simulink model "assignment_13_force_control_inner_position_2"  (R2022b)
settings: Solver=VariableStepAuto  StartTime=0.0  StopTime=5  RelTol=1e-3
values from neighbouring files (symbols this model uses):
  dq0 = [0;0;0]    [assignment_10.m]    (also in assignment_11.m; assignment_12.m; assignment_13.m; assignment_6.m)
  Fd = [0; 0; 3]    [assignment_13.m]
  K_env = 1000    [assignment_11.m]    (also in assignment_12.m = 100; assignment_13.m = 100)
  Kd_pos = 10    [assignment_13.m]
  Ki_force = 0.1    [assignment_13.m]
  Kp_force = 1    [assignment_13.m]
  Kp_pos = 10    [assignment_13.m]
  q0 = [0;0;0]    [assignment_10.m]    (also in assignment_11.m; assignment_12.m; assignment_13.m = [0; pi/2; -pi/2]; assignment_6.m)
  x_home = direct_kinematics(q_home)    [assignment_11.m]    (also in assignment_13.m = x_home(1:3, 1))
  x_ref = x_rest_env    [assignment_13.m]
  x_rest_env = direct_kinematics(q_rest_env)    [assignment_11.m]    (also in assignment_12.m; assignment_13.m = x_rest_env(1:3, 1))
settings Model: Creator=acesi  LastModifiedBy=Manu

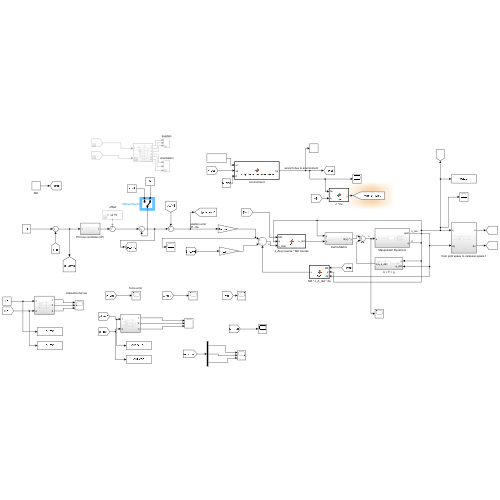
[thumbnail: Simulink's stored preview of the top-level diagram]
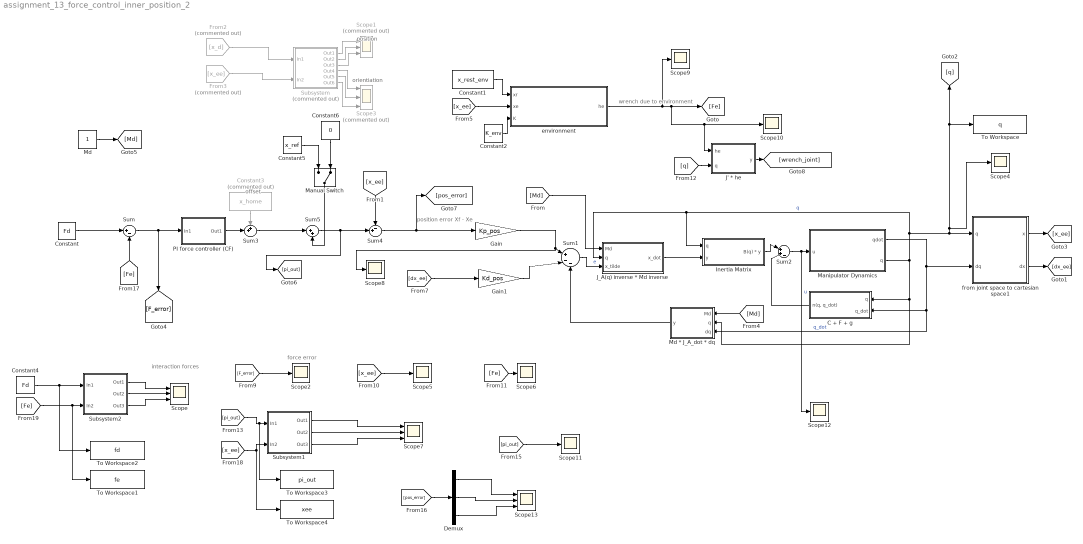
== system assignment_13_force_control_inner_position_2 ==
  note: force error
  note: interaction forces
  note: position error
      | Xf - Xe
  note: offset
  note: orientiation
  note: position
  note: wrench due to environment
  C + F + g : Subsystem
  Constant : Constant  Value=Fd
  Constant1 : Constant  Value=x_rest_env
  Constant2 : Constant  Value=K_env
  Constant3 : Constant  Commented=on  Value=x_home
  Constant4 : Constant  Value=Fd
  Constant5 : Constant  Value=x_ref
  Constant6 : Constant  Value=0
  Demux : Demux  Outputs=3
  From2 : From  Commented=on  GotoTag=x_d
  From3 : From  Commented=on  GotoTag=x_ee
  Gain : Gain  Gain=Kp_pos
  Gain1 : Gain  Gain=Kd_pos
  Inertia Matrix : Subsystem
  J' * he : MATLAB Function  TreatAsAtomicUnit=on
  J_A(q) inverse * Md inverse : MATLAB Function  TreatAsAtomicUnit=on
  Manipulator Dynamics : Subsystem
  Manual Switch : ManualSwitch  CurrentSetting=0
  Md : Constant
  Md * J_A_dot * dq : MATLAB Function  TreatAsAtomicUnit=on
  PI force controller (CF) : Subsystem
  Scope : Scope  NumInputPorts=3
  Scope1 : Scope  Commented=on  NumInputPorts=3
  Scope{2,4..6,8..12} (9 alike) : Scope
  Scope13 : Scope  NumInputPorts=3
  Scope3 : Scope  Commented=on  NumInputPorts=3
  Scope7 : Scope  NumInputPorts=3
  Subsystem : Subsystem  Commented=on
  Subsystem1 : Subsystem
  Subsystem2 : Subsystem
  Sum : Sum  Inputs=|+-
  Sum1 : Sum  Inputs=|+--
  Sum2 : Sum  Inputs=|++-
  Sum3 : Sum  Inputs=++|
  Sum4 : Sum  Inputs=-+|
  Sum5 : Sum  Inputs=|++
  To Workspace : ToWorkspace  VariableName=q  SaveFormat=Timeseries  SampleTime=-1
  To Workspace1 : ToWorkspace  VariableName=fe  SaveFormat=Timeseries  SampleTime=-1
  To Workspace2 : ToWorkspace  VariableName=fd  SaveFormat=Timeseries  SampleTime=-1
  To Workspace3 : ToWorkspace  VariableName=pi_out  SaveFormat=Timeseries  SampleTime=-1
  To Workspace4 : ToWorkspace  VariableName=xee  SaveFormat=Timeseries  SampleTime=-1
  environment : MATLAB Function  TreatAsAtomicUnit=on
  from joint space to cartesian space1 : Subsystem
  wires:
  Manipulator Dynamics/1(qdot) -> from joint space to cartesian space1/2(dq), Md * J_A_dot * dq/3(dq), C + F + g/2(q_dot)  "q_dot"
  Manipulator Dynamics/2(q) -> J_A(q) inverse * Md inverse/2(q), Inertia Matrix/1(q), from joint space to cartesian space1/1(q), Scope4/1, To Workspace/1, [q], Md * J_A_dot * dq/2(q), C + F + g/1(q)  "q"
  Inertia Matrix/1(B(q) * y) -> Sum2/1
  Sum2/1 -> Scope12/1, Manipulator Dynamics/1(u)  "u"
  C + F + g/1("n(q, q_dot)") -> Sum2/2
  Sum1/1 -> J_A(q) inverse * Md inverse/3(x_tilde)  "e"
  J_A(q) inverse * Md inverse/1(x_dot) -> Inertia Matrix/2(y)
  From2/1 -> Subsystem/1(In1)
  From3/1 -> Subsystem/2(In2)
  Subsystem/6(Out6) -> Scope3/3
  Subsystem/2(Out2) -> Scope1/2
  Subsystem/4(Out4) -> Scope3/1
  Subsystem/3(Out3) -> Scope1/3
  Subsystem/5(Out5) -> Scope3/2
  Subsystem/1(Out1) -> Scope1/1
  [Md] -> J_A(q) inverse * Md inverse/1(Md)
  Md/1 -> [Md]
  [Md] -> Md * J_A_dot * dq/1(Md)
  Constant2/1 -> environment/3(K)
  [x_ee] -> environment/2(xe)
  Constant1/1 -> environment/1(xr)
  environment/1(he) -> Scope9/1, Scope10/1, J' * he/1(he), [Fe]
  from joint space to cartesian space1/1(x) -> [x_ee]
  from joint space to cartesian space1/2(dx) -> [dx_ee]
  PI force controller (CF)/1(Out1) -> Sum3/2
  Sum/1 -> PI force controller (CF)/1(In1), [F_error]
  [x_ee] -> Sum4/1
  Sum4/1 -> [pos_error], Gain/1
  Md * J_A_dot * dq/1(y) -> Sum1/3
  [Fe] -> Sum/2
  [F_error] -> Scope2/1
  [x_ee] -> Scope5/1
  [dx_ee] -> Gain1/1
  Gain1/1 -> Sum1/2
  [Fe] -> Scope6/1
  [q] -> J' * he/2(q)
  Gain/1 -> Scope8/1, Sum1/1
  [pi_out] -> To Workspace3/1, Subsystem1/1(In1)
  Subsystem1/1(Out1) -> Scope7/1
  [x_ee] -> To Workspace4/1, Subsystem1/2(In2)
  Subsystem1/2(Out2) -> Scope7/2
  Subsystem1/3(Out3) -> Scope7/3
  [pi_out] -> Scope11/1
  J' * he/1(y) -> [wrench_joint]
  Demux/3 -> Scope13/3
  Demux/1 -> Scope13/1
  [pos_error] -> Demux/1
  Demux/2 -> Scope13/2
  Sum3/1 -> Sum5/1
  [Fe] -> Subsystem2/2(In2), To Workspace1/1
  Constant4/1 -> Subsystem2/1(In1), To Workspace2/1
  Subsystem2/1(Out1) -> Scope/1
  Subsystem2/2(Out2) -> Scope/2
  Subsystem2/3(Out3) -> Scope/3
  Constant/1 -> Sum/1
  Constant3/1 -> Sum3/1
  Constant5/1 -> Manual Switch/1
  Constant6/1 -> Manual Switch/2
  Sum5/1 -> [pi_out], Sum4/2
  Manual Switch/1 -> Sum5/2

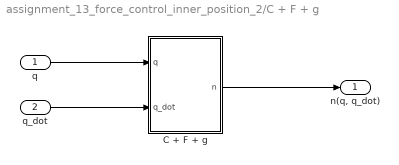
== system assignment_13_force_control_inner_position_2/C + F + g ==
  q : Inport
  q_dot : Inport  Port=2
  C + F + g : MATLAB Function  TreatAsAtomicUnit=on
  "n(q, q_dot)" : Outport
  wires:
  C + F + g/1(n) -> "n(q, q_dot)"/1
  q/1 -> C + F + g/1(q)
  q_dot/1 -> C + F + g/2(q_dot)

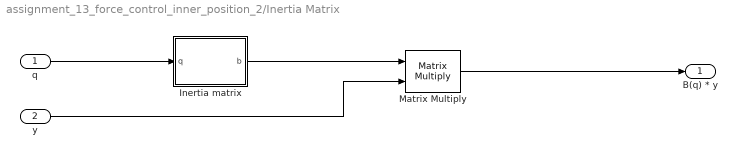
== system assignment_13_force_control_inner_position_2/Inertia Matrix ==
  q : Inport
  y : Inport  Port=2
  Inertia matrix : MATLAB Function  TreatAsAtomicUnit=on
  Matrix Multiply : Product  Multiplication=Matrix(*)
  B(q) * y : Outport
  wires:
  q/1 -> Inertia matrix/1(q)
  Inertia matrix/1(b) -> Matrix Multiply/1
  y/1 -> Matrix Multiply/2
  Matrix Multiply/1 -> B(q) * y/1

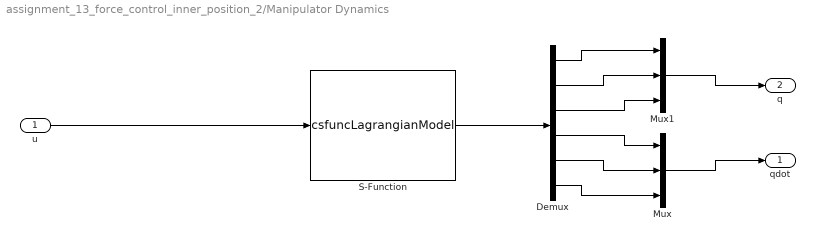
== system assignment_13_force_control_inner_position_2/Manipulator Dynamics ==
  u : Inport
  Demux : Demux  Outputs=6
  Mux : Mux  Inputs=3
  Mux1 : Mux  Inputs=3
  S-Function : S-Function  FunctionName=csfuncLagrangianModel  Parameters=q0 dq0  SFunctionDeploymentMode=off  EnableBusSupport=off
  qdot : Outport
  q : Outport  Port=2
  wires:
  u/1 -> S-Function/1
  S-Function/1 -> Demux/1
  Mux1/1 -> q/1
  Mux/1 -> qdot/1
  Demux/6 -> Mux/3
  Demux/5 -> Mux/2
  Demux/4 -> Mux/1
  Demux/3 -> Mux1/3
  Demux/2 -> Mux1/2
  Demux/1 -> Mux1/1

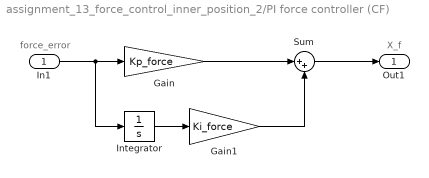
== system assignment_13_force_control_inner_position_2/PI force controller (CF) ==
  note: X_f
  note: force_error
  In1 : Inport
  Gain : Gain  Gain=Kp_force
  Gain1 : Gain  Gain=Ki_force
  Integrator : Integrator
  Sum : Sum  Inputs=|++
  Out1 : Outport
  wires:
  In1/1 -> Integrator/1, Gain/1
  Sum/1 -> Out1/1
  Gain/1 -> Sum/1
  Gain1/1 -> Sum/2
  Integrator/1 -> Gain1/1

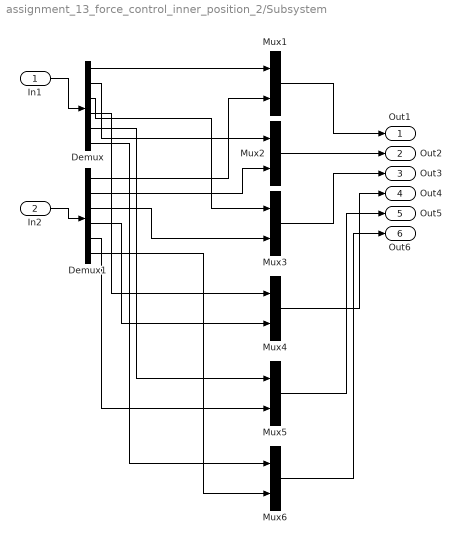
== system assignment_13_force_control_inner_position_2/Subsystem ==
  In1 : Inport
  In2 : Inport  Port=2
  Demux : Demux  Outputs=6
  Demux1 : Demux  Outputs=6
  Mux{1..6} (6 alike) : Mux  Inputs=2
  Out1 : Outport
  Out2 : Outport  Port=2
  Out3 : Outport  Port=3
  Out4 : Outport  Port=4
  Out5 : Outport  Port=5
  Out6 : Outport  Port=6
  wires:
  Demux/1 -> Mux1/1
  Demux/3 -> Mux3/1
  Demux/2 -> Mux2/1
  Demux1/1 -> Mux1/2
  Mux2/1 -> Out2/1
  Demux1/3 -> Mux3/2
  Demux1/2 -> Mux2/2
  Mux3/1 -> Out3/1
  Mux1/1 -> Out1/1
  In2/1 -> Demux1/1
  In1/1 -> Demux/1
  Demux1/4 -> Mux4/2
  Demux/4 -> Mux4/1
  Demux/5 -> Mux5/1
  Demux1/5 -> Mux5/2
  Demux/6 -> Mux6/1
  Demux1/6 -> Mux6/2
  Mux4/1 -> Out4/1
  Mux5/1 -> Out5/1
  Mux6/1 -> Out6/1

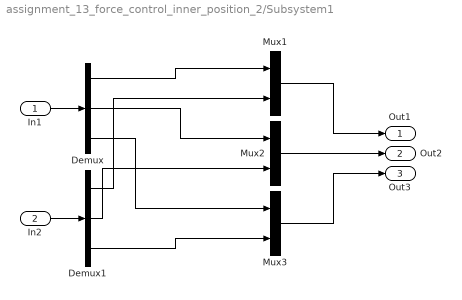
== system assignment_13_force_control_inner_position_2/Subsystem1 ==
  In1 : Inport
  In2 : Inport  Port=2
  Demux : Demux  Outputs=3
  Demux1 : Demux  Outputs=3
  Mux1 : Mux  Inputs=2
  Mux2 : Mux  Inputs=2
  Mux3 : Mux  Inputs=2
  Out1 : Outport
  Out2 : Outport  Port=2
  Out3 : Outport  Port=3
  wires:
  Mux2/1 -> Out2/1
  Mux3/1 -> Out3/1
  Mux1/1 -> Out1/1
  In2/1 -> Demux1/1
  In1/1 -> Demux/1
  Demux/1 -> Mux1/1
  Demux/2 -> Mux2/1
  Demux/3 -> Mux3/1
  Demux1/1 -> Mux1/2
  Demux1/2 -> Mux2/2
  Demux1/3 -> Mux3/2

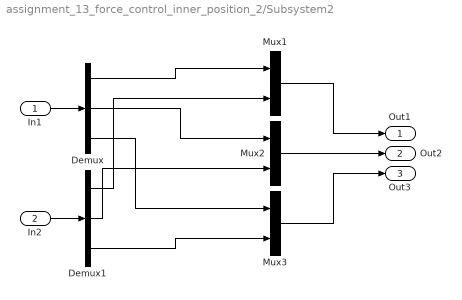
== system assignment_13_force_control_inner_position_2/Subsystem2 ==
  In1 : Inport
  In2 : Inport  Port=2
  Demux : Demux  Outputs=3
  Demux1 : Demux  Outputs=3
  Mux1 : Mux  Inputs=2
  Mux2 : Mux  Inputs=2
  Mux3 : Mux  Inputs=2
  Out1 : Outport
  Out2 : Outport  Port=2
  Out3 : Outport  Port=3
  wires:
  Mux2/1 -> Out2/1
  Mux3/1 -> Out3/1
  Mux1/1 -> Out1/1
  In2/1 -> Demux1/1
  In1/1 -> Demux/1
  Demux/1 -> Mux1/1
  Demux/2 -> Mux2/1
  Demux/3 -> Mux3/1
  Demux1/1 -> Mux1/2
  Demux1/2 -> Mux2/2
  Demux1/3 -> Mux3/2

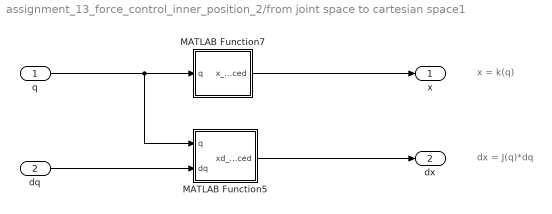
== system assignment_13_force_control_inner_position_2/from joint space to cartesian space1 ==
  note: dx = J(q)*dq
  note: x = k(q)
  q : Inport
  dq : Inport  Port=2
  MATLAB Function5 : MATLAB Function  TreatAsAtomicUnit=on
  MATLAB Function7 : MATLAB Function  TreatAsAtomicUnit=on
  x : Outport
  dx : Outport  Port=2
  wires:
  q/1 -> MATLAB Function5/1(q), MATLAB Function7/1(q)
  MATLAB Function7/1(x_reduced) -> x/1
  MATLAB Function5/1(xd_reduced) -> dx/1
  dq/1 -> MATLAB Function5/2(dq)

== matlab function assignment_13_force_control_inner_position_2/C + F + g/C + F + g ==
  data: q input; n output; q_dot input
function n = N(q, q_dot)
    % return n = C(q, qd) + F + g(q) 

    g = get_G_hardcoded(q);
    c = get_C_hardcoded(q, q_dot) * q_dot;

    n = g + c;
end

== matlab function assignment_13_force_control_inner_position_2/J_A(q) inverse * Md inverse ==
  data: Md input; q input; x_dot output; x_tilde input
function x_dot = fcn(Md, q, x_tilde)
    J_A = get_JA(q);
    J_A = J_A(1:3, :); % only first 3 rows
   
    x_dot = pinv(J_A) * pinv(Md) * x_tilde;
end

== matlab function assignment_13_force_control_inner_position_2/J' * he ==
  data: he input; y output; q input
function y = fcn(he, q)
% maps wrench to joint space (qual'è la nomenclatura corretta?)
J_G = get_JG(q); 
y_ = J_G(1:3, :)' * he;
y = y_(1:3, 1);

== matlab function assignment_13_force_control_inner_position_2/Md * J_A_dot * dq ==
  data: Md input; q input; y output; dq input
function y = fcn(Md, q, dq)
    J_A_dot = get_JA_dot(q, dq);
    %J_A_dot = J_A_dot(1:3, :); % only first 3 rows

    y_ = Md * J_A_dot * dq;
    y = y_(1:3, 1);
end

== matlab function assignment_13_force_control_inner_position_2/environment ==
  data: xr input; he output; xe input; K input
function he = compute_interaction_force(xr, xe, K)
% xr: rest position of the environment (expressed in the operational space)
% xe: current position of the end effector (expressed in the operational space)
% K: environment spring constant (the env. is modeled as a pure spring)

if xe(3) < xr(3)
    he = zeros(3,1); % no interaction with the environment
else
    % end effector position is larger than the env. rest position
    delta_position = xr - xe;
    he = -K * delta_position; % spring force: f = -kx
    he(1)=0;
    he(2)=0;
end

== matlab function assignment_13_force_control_inner_position_2/from joint space to cartesian space1/MATLAB Function5 ==
  data: q input; dq input; xd_reduced output
function xd_reduced = fun(q, dq)
    Ja = get_JA(q);
    xd = Ja * dq;
    xd_reduced = xd(1:3, 1); 
end

== matlab function assignment_13_force_control_inner_position_2/from joint space to cartesian space1/MATLAB Function7 ==
  data: q input; x_reduced output
function x_reduced = fun(q)
    x = direct_kinematics(q);
    x_reduced = x(1:3, 1);
end

== matlab function assignment_13_force_control_inner_position_2/Inertia Matrix/Inertia matrix ==
  data: q input; b output
function b = B(q)

    b = get_B_hardcoded(q);

end
